simulink model "double_pendulum"  (R2019b)
settings: Solver=VariableStepAuto  StartTime=0.0  StopTime=7  MaxStep=0.01  RelTol=1e-3
values from neighbouring files (symbols this model uses):
  A = [0 1 0 0 0 0 ... (first row only)    [models_lqr_pole_placement.m]
  B = [0 ... (first row only)    [models_lqr_pole_placement.m]
  C = eye(6)    [models_lqr_pole_placement.m]
  D = [0 0 0 ... (first row only)    [h_inf.m]    (also in models_lqr_pole_placement.m = [0])
  K = -Y*inv(P)    [h_inf.m]    (also in models_lqr_pole_placement.m = place(A,B,poles))
  P = solution.parameters    [bvp4c_solution.m]
  w = pi/swing_up_time    [bvp4c_solution.m]
libraries: simulink x9
settings Model: Creator=Wellery  LastModifiedBy=Wellery

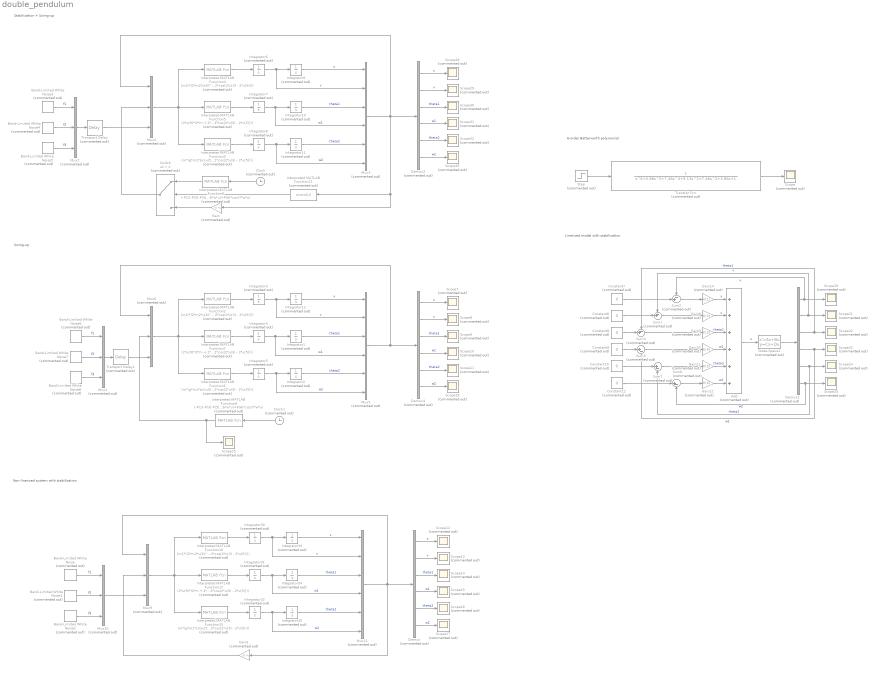
== system double_pendulum ==
  note: Stabilization + Swing-up
  note: 6-order Batterworth polynomial
  note: Linerized model with stabilization
  note: Non-linerized system with stabilization
  note: Swing-up
  Add : Sum  Commented=on  Inputs=++++++
  Band-Limited White Noise : simulink/Sources/Band-Limited White Noise  Commented=on  Cov=[0.015]  Ts=0.1  seed=[23341]
  Band-Limited White Noise1 : simulink/Sources/Band-Limited White Noise  Commented=on  Cov=[0.015]  Ts=0.1  seed=[23341]
  Band-Limited White Noise2 : simulink/Sources/Band-Limited White Noise  Commented=on  Cov=[0.015]  Ts=0.1  seed=[23341]
  Band-Limited White Noise{3..8} (6 alike) : simulink/Sources/Band-Limited White Noise  Commented=on  Cov=[0.01]  Ts=0.1  seed=[23341]
  Clock : Clock  Commented=on
      settings: Decimation=4
  Clock1 : Clock  Commented=on
      settings: Decimation=4
  Constant{6..10,12} (6 alike) : Constant  Commented=on  Value=0
  Demux{,2..4} (4 alike) : Demux  Commented=on  Outputs=6
  Gain : Gain  Commented=on  Gain=-K  Multiplication=Matrix(K*u)
  Gain1 : Gain  Commented=on  Gain=-K  Multiplication=Matrix(K*u)
  Gain10 : Gain  Commented=on  Gain=K(4)
  Gain11 : Gain  Commented=on  Gain=K(5)
  Gain12 : Gain  Commented=on  Gain=K(6)
  Gain14 : Gain  Commented=on  Gain=K(1)
  Gain8 : Gain  Commented=on  Gain=K(2)
  Gain9 : Gain  Commented=on  Gain=K(3)
  Integrator{1..2,10..11} (4 alike) : Integrator  Commented=on  InitialCondition=pi
  Integrator{3..9,12,30..35} (14 alike) : Integrator  Commented=on
  Interpreted MATLAB Function1 : MATLABFcn  Commented=on  MATLABFcn=(m*(g*m1*sin(u(5)) + g*m2*sin(u(5)) - g*m1*sin(2*u(3) - u(5)) - g*m2*sin(2*u(3) - u(5)) + 2*l1*m1*u(4)^2*sin(u(3) - u(5)) + 2*l1*m2*u(4)^2*sin(u(3) - u(5)) + l2*m2*u(6)^2*sin(2*u(3) - 2*u(5))))/(l2*(2*m*m1 + m*m2 + m1*m2 - m1^2*cos(2*u(3)) + m1^2 - m1*m2*cos(2*u(3)) - m*m2*cos(2*u(3) - 2*u(5)))) - (d3*l1*m1^2*u(6) + d3*l1*m2^2*u(6) + d2*l2*m2^2*u(4)*cos(u(3) + u(5)) - d2*l2*m2^2*u(4)*cos(u(3) - u(5)) + 2*d3*l1*m*m1*u(6) + 2*d3*l1*m*m2*u(6) + 2*d3*l1*m1*m2*u(6) - d3*l1*m1^2*u(6)*cos(2*u(3)) - d3*l1*m2^2*u(6)*cos(2*u(3)) + d2*l2*m1*m2*u(4)*cos(u(3) + u(5)) + d1*l1*l2*m2^2*u(2)*cos(2*u(3) - u(5)) - 2*d2*l2*m*m2*u(4)*cos(u(3) - u(5)) - d2*l2*m1*m2*u(4)*cos(u(3) - u(5)) - d1*l1*l2*m2^2*u(2)*cos(u(5)) - 2*d3*l1*m1*m2*u(6)*cos(2*u(3)) + d1*l1*l2*m1*m2*u(2)*cos(2*u(3) - u(5)) - d1*l1*l2*m1*m2*u(2)*cos(u(5)))/(l1*l2^2*m2*(2*m*m1 + m*m2 + m1*m2 - m1^2*cos(2*u(3)) + m1^2 - m1*m2*cos(2*u(3)) - m*m2*cos(2*u(3) - 2*u(5)))) + (u(10)*l1*m1^2 + u(10)*l1*m2^2 - u(9)*l2*m2^2*cos(u(3) - u(5)) + 2*u(10)*l1*m*m1 + 2*u(10)*l1*m*m2 + 2*u(10)*l1*m1*m2 - u(10)*l1*m1^2*cos(2*u(3)) - u(10)*l1*m2^2*cos(2*u(3)) + u(9)*l2*m2^2*cos(u(3) + u(5)) - 2*u(9)*l2*m*m2*cos(u(3) - u(5)) - u(9)*l2*m1*m2*cos(u(3) - u(5)) - u(8)*l1*l2*m2^2*cos(u(5)) - 2*u(10)*l1*m1*m2*cos(2*u(3)) + u(9)*l2*m1*m2*cos(u(3) + u(5)) + u(8)*l1*l2*m2^2*cos(2*u(3) - u(5)) - u(8)*l1*l2*m1*m2*cos(u(5)) + u(8)*l1*l2*m1*m2*cos(2*u(3) - u(5)))/(l1*l2^2*m2*(2*m*m1 + m*m2 + m1*m2 - m1^2*cos(2*u(3)) + m1^2 - m1*m2*cos(2*u(3)) - m*m2*cos(2*u(3) - 2*u(5)))) + (u(7)*(cos(2*u(3) - u(5)) - cos(u(5)))*(m1 + m2))/(l2*(2*m*m1 + m*m2 + m1*m2 - m1^2*cos(2*u(3)) + m1^2 - m1*m2*cos(2*u(3)) - m*m2*cos(2*u(3) - 2*u(5))))
  Interpreted MATLAB Function12 : MATLABFcn  Commented=on  MATLABFcn=norm(u)  OutputDimensions=[1]
  Interpreted MATLAB Function15 : MATLABFcn  Commented=on  MATLABFcn=(m*(g*m1*sin(u(5)) + g*m2*sin(u(5)) - g*m1*sin(2*u(3) - u(5)) - g*m2*sin(2*u(3) - u(5)) + 2*l1*m1*u(4)^2*sin(u(3) - u(5)) + 2*l1*m2*u(4)^2*sin(u(3) - u(5)) + l2*m2*u(6)^2*sin(2*u(3) - 2*u(5))))/(l2*(2*m*m1 + m*m2 + m1*m2 - m1^2*cos(2*u(3)) + m1^2 - m1*m2*cos(2*u(3)) - m*m2*cos(2*u(3) - 2*u(5)))) - (d3*l1*m1^2*u(6) + d3*l1*m2^2*u(6) + d2*l2*m2^2*u(4)*cos(u(3) + u(5)) - d2*l2*m2^2*u(4)*cos(u(3) - u(5)) + 2*d3*l1*m*m1*u(6) + 2*d3*l1*m*m2*u(6) + 2*d3*l1*m1*m2*u(6) - d3*l1*m1^2*u(6)*cos(2*u(3)) - d3*l1*m2^2*u(6)*cos(2*u(3)) + d2*l2*m1*m2*u(4)*cos(u(3) + u(5)) + d1*l1*l2*m2^2*u(2)*cos(2*u(3) - u(5)) - 2*d2*l2*m*m2*u(4)*cos(u(3) - u(5)) - d2*l2*m1*m2*u(4)*cos(u(3) - u(5)) - d1*l1*l2*m2^2*u(2)*cos(u(5)) - 2*d3*l1*m1*m2*u(6)*cos(2*u(3)) + d1*l1*l2*m1*m2*u(2)*cos(2*u(3) - u(5)) - d1*l1*l2*m1*m2*u(2)*cos(u(5)))/(l1*l2^2*m2*(2*m*m1 + m*m2 + m1*m2 - m1^2*cos(2*u(3)) + m1^2 - m1*m2*cos(2*u(3)) - m*m2*cos(2*u(3) - 2*u(5)))) + (u(10)*l1*m1^2 + u(10)*l1*m2^2 - u(9)*l2*m2^2*cos(u(3) - u(5)) + 2*u(10)*l1*m*m1 + 2*u(10)*l1*m*m2 + 2*u(10)*l1*m1*m2 - u(10)*l1*m1^2*cos(2*u(3)) - u(10)*l1*m2^2*cos(2*u(3)) + u(9)*l2*m2^2*cos(u(3) + u(5)) - 2*u(9)*l2*m*m2*cos(u(3) - u(5)) - u(9)*l2*m1*m2*cos(u(3) - u(5)) - u(8)*l1*l2*m2^2*cos(u(5)) - 2*u(10)*l1*m1*m2*cos(2*u(3)) + u(9)*l2*m1*m2*cos(u(3) + u(5)) + u(8)*l1*l2*m2^2*cos(2*u(3) - u(5)) - u(8)*l1*l2*m1*m2*cos(u(5)) + u(8)*l1*l2*m1*m2*cos(2*u(3) - u(5)))/(l1*l2^2*m2*(2*m*m1 + m*m2 + m1*m2 - m1^2*cos(2*u(3)) + m1^2 - m1*m2*cos(2*u(3)) - m*m2*cos(2*u(3) - 2*u(5)))) + (u(7)*(cos(2*u(3) - u(5)) - cos(u(5)))*(m1 + m2))/(l2*(2*m*m1 + m*m2 + m1*m2 - m1^2*cos(2*u(3)) + m1^2 - m1*m2*cos(2*u(3)) - m*m2*cos(2*u(3) - 2*u(5))))
  Interpreted MATLAB Function16 : MATLABFcn  Commented=on  MATLABFcn=(m1*(l2*m2*u(6)^2*sin(2*u(3) - u(5)) - g*m2*sin(2*u(3)) - g*m1*sin(2*u(3)) + 2*l1*m1*u(4)^2*sin(u(3)) + 2*l1*m2*u(4)^2*sin(u(3)) + l2*m2*u(6)^2*sin(u(5))))/(2*m*m1 + m*m2 + m1*m2 - m1^2*cos(2*u(3)) + m1^2 - m1*m2*cos(2*u(3)) - m*m2*cos(2*u(3) - 2*u(5))) + (u(7)*(2*m1 + m2 - m2*cos(2*u(3) - 2*u(5))))/(2*m*m1 + m*m2 + m1*m2 - m1^2*cos(2*u(3)) + m1^2 - m1*m2*cos(2*u(3)) - m*m2*cos(2*u(3) - 2*u(5))) + (u(10)*l1*m1*cos(2*u(3) - u(5)) + u(10)*l1*m2*cos(2*u(3) - u(5)) + 2*u(8)*l1*l2*m1 + u(8)*l1*l2*m2 - 2*u(9)*l2*m1*cos(u(3)) - u(9)*l2*m2*cos(u(3)) - u(10)*l1*m1*cos(u(5)) - u(10)*l1*m2*cos(u(5)) + u(9)*l2*m2*cos(u(3) - 2*u(5)) - u(8)*l1*l2*m2*cos(2*u(3) - 2*u(5)))/(l1*l2*(2*m*m1 + m*m2 + m1*m2 - m1^2*cos(2*u(3)) + m1^2 - m1*m2*cos(2*u(3)) - m*m2*cos(2*u(3) - 2*u(5)))) - (d2*l2*m2*u(4)*cos(u(3) - 2*u(5)) + 2*d1*l1*l2*m1*u(2) + d1*l1*l2*m2*u(2) + d3*l1*m1*u(6)*cos(2*u(3) - u(5)) + d3*l1*m2*u(6)*cos(2*u(3) - u(5)) - 2*d2*l2*m1*u(4)*cos(u(3)) - d2*l2*m2*u(4)*cos(u(3)) - d3*l1*m1*u(6)*cos(u(5)) - d3*l1*m2*u(6)*cos(u(5)) - d1*l1*l2*m2*u(2)*cos(2*u(3) - 2*u(5)))/(l1*l2*(2*m*m1 + m*m2 + m1*m2 - m1^2*cos(2*u(3)) + m1^2 - m1*m2*cos(2*u(3)) - m*m2*cos(2*u(3) - 2*u(5))))
  Interpreted MATLAB Function17 : MATLABFcn  Commented=on  MATLABFcn=(2*u(9)*l2*m + 2*u(9)*l2*m1 + u(9)*l2*m2 + u(10)*l1*m1*cos(u(3) + u(5)) + u(10)*l1*m2*cos(u(3) + u(5)) - 2*u(10)*l1*m*cos(u(3) - u(5)) - u(10)*l1*m1*cos(u(3) - u(5)) - u(10)*l1*m2*cos(u(3) - u(5)) - u(9)*l2*m2*cos(2*u(5)) + u(8)*l1*l2*m2*cos(u(3) - 2*u(5)) - 2*u(8)*l1*l2*m1*cos(u(3)) - u(8)*l1*l2*m2*cos(u(3)))/(l1^2*l2*(2*m*m1 + m*m2 + m1*m2 - m1^2*cos(2*u(3)) + m1^2 - m1*m2*cos(2*u(3)) - m*m2*cos(2*u(3) - 2*u(5)))) - (l1*m1^2*u(4)^2*sin(2*u(3)) - 2*g*m*m1*sin(u(3)) - g*m*m2*sin(u(3)) - 2*g*m1*m2*sin(u(3)) - 2*g*m1^2*sin(u(3)) - g*m*m2*sin(u(3) - 2*u(5)) + l2*m1*m2*u(6)^2*sin(u(3) + u(5)) + 2*l2*m*m2*u(6)^2*sin(u(3) - u(5)) + l2*m1*m2*u(6)^2*sin(u(3) - u(5)) + l1*m1*m2*u(4)^2*sin(2*u(3)) + l1*m*m2*u(4)^2*sin(2*u(3) - 2*u(5)))/(l1*(2*m*m1 + m*m2 + m1*m2 - m1^2*cos(2*u(3)) + m1^2 - m1*m2*cos(2*u(3)) - m*m2*cos(2*u(3) - 2*u(5)))) - (2*d2*l2*m*u(4) + 2*d2*l2*m1*u(4) + d2*l2*m2*u(4) - 2*d3*l1*m*u(6)*cos(u(3) - u(5)) - d3*l1*m1*u(6)*cos(u(3) - u(5)) - d3*l1*m2*u(6)*cos(u(3) - u(5)) - d2*l2*m2*u(4)*cos(2*u(5)) + d3*l1*m1*u(6)*cos(u(3) + u(5)) + d3*l1*m2*u(6)*cos(u(3) + u(5)) - 2*d1*l1*l2*m1*u(2)*cos(u(3)) - d1*l1*l2*m2*u(2)*cos(u(3)) + d1*l1*l2*m2*u(2)*cos(u(3) - 2*u(5)))/(l1^2*l2*(2*m*m1 + m*m2 + m1*m2 - m1^2*cos(2*u(3)) + m1^2 - m1*m2*cos(2*u(3)) - m*m2*cos(2*u(3) - 2*u(5)))) - (u(7)*(2*m1*cos(u(3)) + m2*cos(u(3)) - m2*cos(u(3) - 2*u(5))))/(l1*(2*m*m1 + m*m2 + m1*m2 - m1^2*cos(2*u(3)) + m1^2 - m1*m2*cos(2*u(3)) - m*m2*cos(2*u(3) - 2*u(5))))
  Interpreted MATLAB Function2 : MATLABFcn  Commented=on  MATLABFcn=(m1*(l2*m2*u(6)^2*sin(2*u(3) - u(5)) - g*m2*sin(2*u(3)) - g*m1*sin(2*u(3)) + 2*l1*m1*u(4)^2*sin(u(3)) + 2*l1*m2*u(4)^2*sin(u(3)) + l2*m2*u(6)^2*sin(u(5))))/(2*m*m1 + m*m2 + m1*m2 - m1^2*cos(2*u(3)) + m1^2 - m1*m2*cos(2*u(3)) - m*m2*cos(2*u(3) - 2*u(5))) + (u(7)*(2*m1 + m2 - m2*cos(2*u(3) - 2*u(5))))/(2*m*m1 + m*m2 + m1*m2 - m1^2*cos(2*u(3)) + m1^2 - m1*m2*cos(2*u(3)) - m*m2*cos(2*u(3) - 2*u(5))) + (u(10)*l1*m1*cos(2*u(3) - u(5)) + u(10)*l1*m2*cos(2*u(3) - u(5)) + 2*u(8)*l1*l2*m1 + u(8)*l1*l2*m2 - 2*u(9)*l2*m1*cos(u(3)) - u(9)*l2*m2*cos(u(3)) - u(10)*l1*m1*cos(u(5)) - u(10)*l1*m2*cos(u(5)) + u(9)*l2*m2*cos(u(3) - 2*u(5)) - u(8)*l1*l2*m2*cos(2*u(3) - 2*u(5)))/(l1*l2*(2*m*m1 + m*m2 + m1*m2 - m1^2*cos(2*u(3)) + m1^2 - m1*m2*cos(2*u(3)) - m*m2*cos(2*u(3) - 2*u(5)))) - (d2*l2*m2*u(4)*cos(u(3) - 2*u(5)) + 2*d1*l1*l2*m1*u(2) + d1*l1*l2*m2*u(2) + d3*l1*m1*u(6)*cos(2*u(3) - u(5)) + d3*l1*m2*u(6)*cos(2*u(3) - u(5)) - 2*d2*l2*m1*u(4)*cos(u(3)) - d2*l2*m2*u(4)*cos(u(3)) - d3*l1*m1*u(6)*cos(u(5)) - d3*l1*m2*u(6)*cos(u(5)) - d1*l1*l2*m2*u(2)*cos(2*u(3) - 2*u(5)))/(l1*l2*(2*m*m1 + m*m2 + m1*m2 - m1^2*cos(2*u(3)) + m1^2 - m1*m2*cos(2*u(3)) - m*m2*cos(2*u(3) - 2*u(5))))
  Interpreted MATLAB Function3 : MATLABFcn  Commented=on  MATLABFcn=(m*(g*m1*sin(u(5)) + g*m2*sin(u(5)) - g*m1*sin(2*u(3) - u(5)) - g*m2*sin(2*u(3) - u(5)) + 2*l1*m1*u(4)^2*sin(u(3) - u(5)) + 2*l1*m2*u(4)^2*sin(u(3) - u(5)) + l2*m2*u(6)^2*sin(2*u(3) - 2*u(5))))/(l2*(2*m*m1 + m*m2 + m1*m2 - m1^2*cos(2*u(3)) + m1^2 - m1*m2*cos(2*u(3)) - m*m2*cos(2*u(3) - 2*u(5)))) - (d3*l1*m1^2*u(6) + d3*l1*m2^2*u(6) + d2*l2*m2^2*u(4)*cos(u(3) + u(5)) - d2*l2*m2^2*u(4)*cos(u(3) - u(5)) + 2*d3*l1*m*m1*u(6) + 2*d3*l1*m*m2*u(6) + 2*d3*l1*m1*m2*u(6) - d3*l1*m1^2*u(6)*cos(2*u(3)) - d3*l1*m2^2*u(6)*cos(2*u(3)) + d2*l2*m1*m2*u(4)*cos(u(3) + u(5)) + d1*l1*l2*m2^2*u(2)*cos(2*u(3) - u(5)) - 2*d2*l2*m*m2*u(4)*cos(u(3) - u(5)) - d2*l2*m1*m2*u(4)*cos(u(3) - u(5)) - d1*l1*l2*m2^2*u(2)*cos(u(5)) - 2*d3*l1*m1*m2*u(6)*cos(2*u(3)) + d1*l1*l2*m1*m2*u(2)*cos(2*u(3) - u(5)) - d1*l1*l2*m1*m2*u(2)*cos(u(5)))/(l1*l2^2*m2*(2*m*m1 + m*m2 + m1*m2 - m1^2*cos(2*u(3)) + m1^2 - m1*m2*cos(2*u(3)) - m*m2*cos(2*u(3) - 2*u(5)))) + (u(10)*l1*m1^2 + u(10)*l1*m2^2 - u(9)*l2*m2^2*cos(u(3) - u(5)) + 2*u(10)*l1*m*m1 + 2*u(10)*l1*m*m2 + 2*u(10)*l1*m1*m2 - u(10)*l1*m1^2*cos(2*u(3)) - u(10)*l1*m2^2*cos(2*u(3)) + u(9)*l2*m2^2*cos(u(3) + u(5)) - 2*u(9)*l2*m*m2*cos(u(3) - u(5)) - u(9)*l2*m1*m2*cos(u(3) - u(5)) - u(8)*l1*l2*m2^2*cos(u(5)) - 2*u(10)*l1*m1*m2*cos(2*u(3)) + u(9)*l2*m1*m2*cos(u(3) + u(5)) + u(8)*l1*l2*m2^2*cos(2*u(3) - u(5)) - u(8)*l1*l2*m1*m2*cos(u(5)) + u(8)*l1*l2*m1*m2*cos(2*u(3) - u(5)))/(l1*l2^2*m2*(2*m*m1 + m*m2 + m1*m2 - m1^2*cos(2*u(3)) + m1^2 - m1*m2*cos(2*u(3)) - m*m2*cos(2*u(3) - 2*u(5)))) + (u(7)*(cos(2*u(3) - u(5)) - cos(u(5)))*(m1 + m2))/(l2*(2*m*m1 + m*m2 + m1*m2 - m1^2*cos(2*u(3)) + m1^2 - m1*m2*cos(2*u(3)) - m*m2*cos(2*u(3) - 2*u(5))))
  Interpreted MATLAB Function4 : MATLABFcn  Commented=on  MATLABFcn=(m1*(l2*m2*u(6)^2*sin(2*u(3) - u(5)) - g*m2*sin(2*u(3)) - g*m1*sin(2*u(3)) + 2*l1*m1*u(4)^2*sin(u(3)) + 2*l1*m2*u(4)^2*sin(u(3)) + l2*m2*u(6)^2*sin(u(5))))/(2*m*m1 + m*m2 + m1*m2 - m1^2*cos(2*u(3)) + m1^2 - m1*m2*cos(2*u(3)) - m*m2*cos(2*u(3) - 2*u(5))) + (u(7)*(2*m1 + m2 - m2*cos(2*u(3) - 2*u(5))))/(2*m*m1 + m*m2 + m1*m2 - m1^2*cos(2*u(3)) + m1^2 - m1*m2*cos(2*u(3)) - m*m2*cos(2*u(3) - 2*u(5))) + (u(10)*l1*m1*cos(2*u(3) - u(5)) + u(10)*l1*m2*cos(2*u(3) - u(5)) + 2*u(8)*l1*l2*m1 + u(8)*l1*l2*m2 - 2*u(9)*l2*m1*cos(u(3)) - u(9)*l2*m2*cos(u(3)) - u(10)*l1*m1*cos(u(5)) - u(10)*l1*m2*cos(u(5)) + u(9)*l2*m2*cos(u(3) - 2*u(5)) - u(8)*l1*l2*m2*cos(2*u(3) - 2*u(5)))/(l1*l2*(2*m*m1 + m*m2 + m1*m2 - m1^2*cos(2*u(3)) + m1^2 - m1*m2*cos(2*u(3)) - m*m2*cos(2*u(3) - 2*u(5)))) - (d2*l2*m2*u(4)*cos(u(3) - 2*u(5)) + 2*d1*l1*l2*m1*u(2) + d1*l1*l2*m2*u(2) + d3*l1*m1*u(6)*cos(2*u(3) - u(5)) + d3*l1*m2*u(6)*cos(2*u(3) - u(5)) - 2*d2*l2*m1*u(4)*cos(u(3)) - d2*l2*m2*u(4)*cos(u(3)) - d3*l1*m1*u(6)*cos(u(5)) - d3*l1*m2*u(6)*cos(u(5)) - d1*l1*l2*m2*u(2)*cos(2*u(3) - 2*u(5)))/(l1*l2*(2*m*m1 + m*m2 + m1*m2 - m1^2*cos(2*u(3)) + m1^2 - m1*m2*cos(2*u(3)) - m*m2*cos(2*u(3) - 2*u(5))))
  Interpreted MATLAB Function5 : MATLABFcn  Commented=on  MATLABFcn=(2*u(9)*l2*m + 2*u(9)*l2*m1 + u(9)*l2*m2 + u(10)*l1*m1*cos(u(3) + u(5)) + u(10)*l1*m2*cos(u(3) + u(5)) - 2*u(10)*l1*m*cos(u(3) - u(5)) - u(10)*l1*m1*cos(u(3) - u(5)) - u(10)*l1*m2*cos(u(3) - u(5)) - u(9)*l2*m2*cos(2*u(5)) + u(8)*l1*l2*m2*cos(u(3) - 2*u(5)) - 2*u(8)*l1*l2*m1*cos(u(3)) - u(8)*l1*l2*m2*cos(u(3)))/(l1^2*l2*(2*m*m1 + m*m2 + m1*m2 - m1^2*cos(2*u(3)) + m1^2 - m1*m2*cos(2*u(3)) - m*m2*cos(2*u(3) - 2*u(5)))) - (l1*m1^2*u(4)^2*sin(2*u(3)) - 2*g*m*m1*sin(u(3)) - g*m*m2*sin(u(3)) - 2*g*m1*m2*sin(u(3)) - 2*g*m1^2*sin(u(3)) - g*m*m2*sin(u(3) - 2*u(5)) + l2*m1*m2*u(6)^2*sin(u(3) + u(5)) + 2*l2*m*m2*u(6)^2*sin(u(3) - u(5)) + l2*m1*m2*u(6)^2*sin(u(3) - u(5)) + l1*m1*m2*u(4)^2*sin(2*u(3)) + l1*m*m2*u(4)^2*sin(2*u(3) - 2*u(5)))/(l1*(2*m*m1 + m*m2 + m1*m2 - m1^2*cos(2*u(3)) + m1^2 - m1*m2*cos(2*u(3)) - m*m2*cos(2*u(3) - 2*u(5)))) - (2*d2*l2*m*u(4) + 2*d2*l2*m1*u(4) + d2*l2*m2*u(4) - 2*d3*l1*m*u(6)*cos(u(3) - u(5)) - d3*l1*m1*u(6)*cos(u(3) - u(5)) - d3*l1*m2*u(6)*cos(u(3) - u(5)) - d2*l2*m2*u(4)*cos(2*u(5)) + d3*l1*m1*u(6)*cos(u(3) + u(5)) + d3*l1*m2*u(6)*cos(u(3) + u(5)) - 2*d1*l1*l2*m1*u(2)*cos(u(3)) - d1*l1*l2*m2*u(2)*cos(u(3)) + d1*l1*l2*m2*u(2)*cos(u(3) - 2*u(5)))/(l1^2*l2*(2*m*m1 + m*m2 + m1*m2 - m1^2*cos(2*u(3)) + m1^2 - m1*m2*cos(2*u(3)) - m*m2*cos(2*u(3) - 2*u(5)))) - (u(7)*(2*m1*cos(u(3)) + m2*cos(u(3)) - m2*cos(u(3) - 2*u(5))))/(l1*(2*m*m1 + m*m2 + m1*m2 - m1^2*cos(2*u(3)) + m1^2 - m1*m2*cos(2*u(3)) - m*m2*cos(2*u(3) - 2*u(5))))
  Interpreted MATLAB Function6 : MATLABFcn  Commented=on  MATLABFcn=(-P(1)-P(3)-P(5))+(-P(2)-P(4)-P(6))*cos(w*u)+P(1)*cos(2*w*u)+P(2)*cos(3*w*u)+P(3)*cos(4*w*u)+P(4)*cos(5*w*u)+P(5)*cos(6*w*u)+P(6)*cos(7*w*u)  OutputDimensions=[1]
  Interpreted MATLAB Function7 : MATLABFcn  Commented=on  MATLABFcn=(2*u(9)*l2*m + 2*u(9)*l2*m1 + u(9)*l2*m2 + u(10)*l1*m1*cos(u(3) + u(5)) + u(10)*l1*m2*cos(u(3) + u(5)) - 2*u(10)*l1*m*cos(u(3) - u(5)) - u(10)*l1*m1*cos(u(3) - u(5)) - u(10)*l1*m2*cos(u(3) - u(5)) - u(9)*l2*m2*cos(2*u(5)) + u(8)*l1*l2*m2*cos(u(3) - 2*u(5)) - 2*u(8)*l1*l2*m1*cos(u(3)) - u(8)*l1*l2*m2*cos(u(3)))/(l1^2*l2*(2*m*m1 + m*m2 + m1*m2 - m1^2*cos(2*u(3)) + m1^2 - m1*m2*cos(2*u(3)) - m*m2*cos(2*u(3) - 2*u(5)))) - (l1*m1^2*u(4)^2*sin(2*u(3)) - 2*g*m*m1*sin(u(3)) - g*m*m2*sin(u(3)) - 2*g*m1*m2*sin(u(3)) - 2*g*m1^2*sin(u(3)) - g*m*m2*sin(u(3) - 2*u(5)) + l2*m1*m2*u(6)^2*sin(u(3) + u(5)) + 2*l2*m*m2*u(6)^2*sin(u(3) - u(5)) + l2*m1*m2*u(6)^2*sin(u(3) - u(5)) + l1*m1*m2*u(4)^2*sin(2*u(3)) + l1*m*m2*u(4)^2*sin(2*u(3) - 2*u(5)))/(l1*(2*m*m1 + m*m2 + m1*m2 - m1^2*cos(2*u(3)) + m1^2 - m1*m2*cos(2*u(3)) - m*m2*cos(2*u(3) - 2*u(5)))) - (2*d2*l2*m*u(4) + 2*d2*l2*m1*u(4) + d2*l2*m2*u(4) - 2*d3*l1*m*u(6)*cos(u(3) - u(5)) - d3*l1*m1*u(6)*cos(u(3) - u(5)) - d3*l1*m2*u(6)*cos(u(3) - u(5)) - d2*l2*m2*u(4)*cos(2*u(5)) + d3*l1*m1*u(6)*cos(u(3) + u(5)) + d3*l1*m2*u(6)*cos(u(3) + u(5)) - 2*d1*l1*l2*m1*u(2)*cos(u(3)) - d1*l1*l2*m2*u(2)*cos(u(3)) + d1*l1*l2*m2*u(2)*cos(u(3) - 2*u(5)))/(l1^2*l2*(2*m*m1 + m*m2 + m1*m2 - m1^2*cos(2*u(3)) + m1^2 - m1*m2*cos(2*u(3)) - m*m2*cos(2*u(3) - 2*u(5)))) - (u(7)*(2*m1*cos(u(3)) + m2*cos(u(3)) - m2*cos(u(3) - 2*u(5))))/(l1*(2*m*m1 + m*m2 + m1*m2 - m1^2*cos(2*u(3)) + m1^2 - m1*m2*cos(2*u(3)) - m*m2*cos(2*u(3) - 2*u(5))))
  Interpreted MATLAB Function8 : MATLABFcn  Commented=on  MATLABFcn=(-P(1)-P(3)-P(5))+(-P(2)-P(4)-P(6))*cos(w*u)+P(1)*cos(2*w*u)+P(2)*cos(3*w*u)+P(3)*cos(4*w*u)+P(4)*cos(5*w*u)+P(5)*cos(6*w*u)+P(6)*cos(7*w*u)  OutputDimensions=[1]
  Mux{1..2,4,6,9..10} (6 alike) : Mux  Commented=on  Inputs=3
  Mux11 : Mux  Commented=on  Inputs=6
  Mux3 : Mux  Commented=on  Inputs=6
  Mux5 : Mux  Commented=on  Inputs=6
  Scope{,7..25,28..33} (26 alike) : Scope  Commented=on
  State-Space1 : StateSpace  Commented=on  A=A  B=B  C=C  D=D  InitialCondition=[0 0 0.1 0 0 0]
  Step : Step  Commented=on  SampleTime=0
  Sum1 : Sum  Commented=on  Inputs=-+|
  Sum2 : Sum  Commented=on  Inputs=-+|
  Sum3 : Sum  Commented=on  Inputs=-+|
  Sum5 : Sum  Commented=on  Inputs=|+-
  Sum6 : Sum  Commented=on  Inputs=|+-
  Sum7 : Sum  Commented=on  Inputs=|+-
  Switch : Switch  Commented=on  Criteria=u2 > Threshold  Threshold=2
  Transfer Fcn : TransferFcn  Commented=on  Denominator=[1 3.86 7.46 9.13 7.46 3.86 1]
  Transport Delay : TransportDelay  Commented=on  DelayTime=3
  Transport Delay1 : TransportDelay  Commented=on  DelayTime=4
  wires:
  Add/1 -> State-Space1/1  "u"
  Band-Limited White Noise/1 -> Mux10/1  "f1"
  Band-Limited White Noise1/1 -> Mux10/2  "f2"
  Band-Limited White Noise2/1 -> Mux10/3  "f3"
  Interpreted MATLAB Function17/1 -> Integrator31/1
  Mux9/1 -> Interpreted MATLAB Function17/1, Interpreted MATLAB Function15/1, Interpreted MATLAB Function16/1
  Interpreted MATLAB Function16/1 -> Integrator30/1
  Interpreted MATLAB Function15/1 -> Integrator32/1
  Integrator30/1 -> Mux11/2, Integrator33/1  "v"
  Integrator31/1 -> Mux11/4, Integrator34/1  "w1"
  Integrator32/1 -> Mux11/6, Integrator35/1  "w2"
  Integrator33/1 -> Mux11/1  "x"
  Integrator34/1 -> Mux11/3  "theta1"
  Integrator35/1 -> Mux11/5  "theta2"
  Mux11/1 -> Demux/1, Mux9/1, Gain1/1
  Demux/1 -> Scope12/1  "x"
  Demux/2 -> Scope13/1  "v"
  Demux/3 -> Scope14/1  "theta1"
  Demux/4 -> Scope15/1  "w1"
  Demux/5 -> Scope16/1  "theta2"
  Demux/6 -> Scope17/1  "w2"
  Constant7/1 -> Sum2/2
  State-Space1/1 -> Demux2/1
  Demux2/6 -> Sum6/2, Scope20/1  "w2"
  Demux2/5 -> Sum7/2, Scope24/1  "theta2"
  Demux2/1 -> Scope19/1, Sum2/1  "x"
  Demux2/2 -> Sum1/1, Scope21/1  "v"
  Demux2/3 -> Sum3/1, Scope22/1  "theta1"
  Demux2/4 -> Scope23/1, Sum5/2  "w1"
  Constant6/1 -> Sum1/2
  Constant8/1 -> Sum3/2
  Constant9/1 -> Sum5/1
  Sum2/1 -> Gain14/1
  Sum1/1 -> Gain8/1
  Sum3/1 -> Gain9/1
  Sum6/1 -> Gain12/1
  Gain14/1 -> Add/1  "x"
  Gain8/1 -> Add/2  "v"
  Gain9/1 -> Add/3  "theta1"
  Gain10/1 -> Add/4  "w1"
  Gain11/1 -> Add/5  "theta2"
  Gain12/1 -> Add/6  "w2"
  Constant12/1 -> Sum6/1
  Sum7/1 -> Gain11/1
  Constant10/1 -> Sum7/1
  Sum5/1 -> Gain10/1
  Step/1 -> Transfer Fcn/1
  Transfer Fcn/1 -> Scope/1
  Integrator7/1 -> Mux3/4, Integrator10/1  "w1"
  Interpreted MATLAB Function3/1 -> Integrator8/1
  Mux4/1 -> Interpreted MATLAB Function5/1, Interpreted MATLAB Function3/1, Interpreted MATLAB Function4/1
  Demux3/4 -> Scope31/1  "w1"
  Band-Limited White Noise3/1 -> Mux2/1  "f1"
  Interpreted MATLAB Function4/1 -> Integrator6/1
  Band-Limited White Noise5/1 -> Mux2/3  "f3"
  Demux3/3 -> Scope30/1  "theta1"
  Integrator9/1 -> Mux3/1  "x"
  Demux3/1 -> Scope28/1  "x"
  Integrator10/1 -> Mux3/3  "theta1"
  Mux3/1 -> Interpreted MATLAB Function12/1, Gain/1, Demux3/1, Mux4/1
  Demux3/6 -> Scope33/1  "w2"
  Demux3/2 -> Scope29/1  "v"
  Integrator6/1 -> Mux3/2, Integrator9/1  "v"
  Integrator11/1 -> Mux3/5  "theta2"
  Integrator8/1 -> Mux3/6, Integrator11/1  "w2"
  Band-Limited White Noise4/1 -> Mux2/2  "f2"
  Interpreted MATLAB Function5/1 -> Integrator7/1
  Demux3/5 -> Scope32/1  "theta2"
  Clock/1 -> Interpreted MATLAB Function6/1
  Mux10/1 -> Mux9/3
  Mux2/1 -> Transport Delay/1
  Gain1/1 -> Mux9/2
  Switch/1 -> Mux4/2
  Transport Delay/1 -> Mux4/3
  Interpreted MATLAB Function7/1 -> Integrator4/1
  Transport Delay1/1 -> Mux6/3
  Integrator3/1 -> Mux5/2, Integrator12/1  "v"
  Band-Limited White Noise7/1 -> Mux1/2  "f2"
  Demux4/5 -> Scope11/1  "theta2"
  Demux4/6 -> Scope18/1  "w2"
  Band-Limited White Noise8/1 -> Mux1/3  "f3"
  Integrator4/1 -> Mux5/4, Integrator1/1  "w1"
  Mux6/1 -> Interpreted MATLAB Function7/1, Interpreted MATLAB Function1/1, Interpreted MATLAB Function2/1
  Interpreted MATLAB Function1/1 -> Integrator5/1
  Integrator1/1 -> Mux5/3  "theta1"
  Band-Limited White Noise6/1 -> Mux1/1  "f1"
  Demux4/4 -> Scope10/1  "w1"
  Demux4/1 -> Scope7/1  "x"
  Mux5/1 -> Demux4/1, Mux6/1
  Interpreted MATLAB Function2/1 -> Integrator3/1
  Demux4/3 -> Scope9/1  "theta1"
  Integrator5/1 -> Mux5/6, Integrator2/1  "w2"
  Clock1/1 -> Interpreted MATLAB Function8/1
  Demux4/2 -> Scope8/1  "v"
  Integrator12/1 -> Mux5/1  "x"
  Mux1/1 -> Transport Delay1/1
  Interpreted MATLAB Function8/1 -> Scope25/1, Mux6/2
  Integrator2/1 -> Mux5/5  "theta2"
  Interpreted MATLAB Function12/1 -> Switch/2
  Interpreted MATLAB Function6/1 -> Switch/1
  Gain/1 -> Switch/3
